simulink model "EZQStEnCtrl"  (R2018b)
settings: Solver=FixedStepDiscrete  StartTime=0.0  StopTime=10.0  FixedStep=0.01  RelTol=1e-3
undefined symbols (not defined in the file or in its folder): data, DrvStFtEn_Clear, DrvStFtEn_Set, PassStFtEn_Clear, PassStFtEn_Set, SecRwLtStArmScrnEn_Clear, SecRwLtStArmScrnEn_Set, SecRwLtStBkReclnEn_Clear, SecRwLtStBkReclnEn_Set, SecRwLtStFwdBkwdEn_Clear, SecRwLtStFwdBkwdEn_Set, SecRwLtStLgrstUpwdDnwdEn_Clear, SecRwLtStLgrstUpwdDnwdEn_Set, SecRwLtStLtwdRtwdEn_Clear, SecRwLtStLtwdRtwdEn_Set, SecRwRtStArmScrnEn_Clear, SecRwRtStArmScrnEn_Set, SecRwRtStBkReclnEn_Clear, SecRwRtStBkReclnEn_Set, SecRwRtStFwdBkwdEn_Clear, SecRwRtStFwdBkwdEn_Set, SecRwRtStLgrstUpwdDnwdEn_Clear, SecRwRtStLgrstUpwdDnwdEn_Set, SecRwRtStLtwdRtwdEn_Clear, SecRwRtStLtwdRtwdEn_Set
libraries: simulink x1
settings Model: Creator=sn2xws  LastModifiedBy=sn2xws
settings DataIOCC: SaveFormat=StructureWithTime
settings OptimizationCC: DefaultParameterBehavior=Inlined  EnhancedBackFolding=on  PassReuseOutputArgsAs=Individual arguments  ZeroExternalMemoryAtStartup=off  ZeroInternalMemoryAtStartup=off  OptimizeBlockOrder=speed  DifferentSizesBufferReuse=on  OptimizationCustomize=off
settings DebuggingCC: ParameterTunabilityLossMsg=error
settings ModelReferenceCC: ModelReferenceNumInstancesAllowed=Single
settings SFSimCC: MATLABDynamicMemAlloc=off
settings RTWCC: SystemTargetFile=autosar.tlc  GenCodeOnly=on  TemplateMakefile=ert_default_tmf  Description=AUTOSAR  GenerateReport=on  IncludeHyperlinkInReport=on  LaunchReport=on  GenerateTraceInfo=on  GenerateTraceReport=on  GenerateTraceReportSl=on  GenerateTraceReportSf=on  GenerateTraceReportEml=on  GenerateCodeMetricsReport=on
settings CodeAppCC: ForceParamTrailComments=on  IgnoreCustomStorageClasses=off  OperatorAnnotations=on  SimulinkDataObjDesc=on  SFDataObjDesc=on  InsertBlockDesc=on
settings STFCustomTargetCC: TargetLangStandard=C99 (ISO)  MultiwordLength=256  ParMdlRefBuildCompliant=on  CompOptLevelCompliant=on  IncludeMdlTerminateFcn=off  CombineOutputUpdateFcns=on  SuppressErrorStatus=on  ERTCustomFileBanners=on  SupportNonFinite=off  SupportComplex=off  SupportContinuousTime=off  SupportNonInlinedSFcns=off  RemoveResetFunc=on  MATLABClassNameForMDSCustomization=Simulink.SoftwareTarget.ERTCustomization  AutosarCompliant=on  UseToolchainInfoCompliant=on  LookupTableObjectStructAxisOrder=2,1,3,4,...  LUTObjectStructOrderEvenSpacing=Size,Table,Breakpoints  SystemTargetFile=autosar.tlc
settings ERTTargetCC: TargetLangStandard=C99 (ISO)  ConcurrentExecutionCompliant=off  IncludeMdlTerminateFcn=off  SuppressErrorStatus=on  SupportNonFinite=off  SupportComplex=off  ModelStepFunctionPrototypeControlCompliant=off  CPPClassGenCompliant=off  AutosarCompliant=on  LookupTableObjectStructAxisOrder=2,1,3,4,...  LUTObjectStructOrderEvenSpacing=Size,Table,Breakpoints  InlinedParameterPlacement=NonHierarchical  ERTCustomFileTemplate=example_file_process.tlc  ERTFilePackagingFormat=Compact

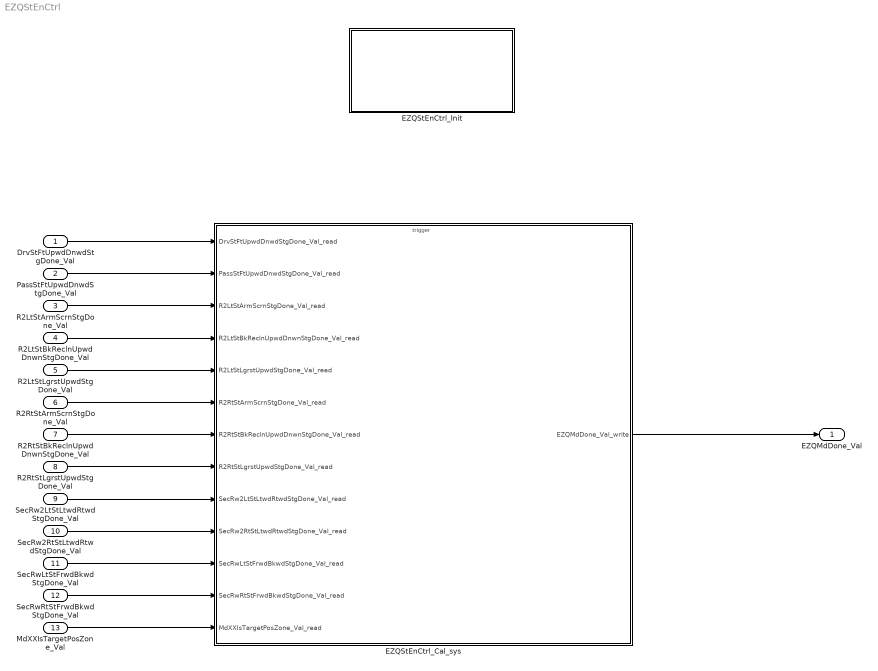
== system EZQStEnCtrl ==
  DrvStFtUpwdDnwdStgDone_Val : Inport  OutDataTypeStr=boolean  PortDimensions=1
  PassStFtUpwdDnwdStgDone_Val : Inport  Port=2  OutDataTypeStr=boolean  PortDimensions=1
  R2LtStArmScrnStgDone_Val : Inport  Port=3  OutDataTypeStr=boolean  PortDimensions=1
  R2LtStBkReclnUpwdDnwnStgDone_Val : Inport  Port=4  OutDataTypeStr=boolean  PortDimensions=1
  R2LtStLgrstUpwdStgDone_Val : Inport  Port=5  OutDataTypeStr=boolean  PortDimensions=1
  R2RtStArmScrnStgDone_Val : Inport  Port=6  OutDataTypeStr=boolean  PortDimensions=1
  R2RtStBkReclnUpwdDnwnStgDone_Val : Inport  Port=7  OutDataTypeStr=boolean  PortDimensions=1
  R2RtStLgrstUpwdStgDone_Val : Inport  Port=8  OutDataTypeStr=boolean  PortDimensions=1
  SecRw2LtStLtwdRtwdStgDone_Val : Inport  Port=9  OutDataTypeStr=boolean  PortDimensions=1
  SecRw2RtStLtwdRtwdStgDone_Val : Inport  Port=10  OutDataTypeStr=boolean  PortDimensions=1
  SecRwLtStFrwdBkwdStgDone_Val : Inport  Port=11  OutDataTypeStr=boolean  PortDimensions=1
  SecRwRtStFrwdBkwdStgDone_Val : Inport  Port=12  OutDataTypeStr=boolean  PortDimensions=1
  MdXXIsTargetPosZone_Val : Inport  Port=13  OutDataTypeStr=uint32  PortDimensions=1
  EZQStEnCtrl_Cal_sys : Subsystem
  EZQStEnCtrl_Init : Subsystem
  EZQMdDone_Val : Outport  OutDataTypeStr=uint8  PortDimensions=1
  wires:
  DrvStFtUpwdDnwdStgDone_Val/1 -> EZQStEnCtrl_Cal_sys/1(DrvStFtUpwdDnwdStgDone_Val_read)
  PassStFtUpwdDnwdStgDone_Val/1 -> EZQStEnCtrl_Cal_sys/2(PassStFtUpwdDnwdStgDone_Val_read)
  R2LtStArmScrnStgDone_Val/1 -> EZQStEnCtrl_Cal_sys/3(R2LtStArmScrnStgDone_Val_read)
  R2LtStBkReclnUpwdDnwnStgDone_Val/1 -> EZQStEnCtrl_Cal_sys/4(R2LtStBkReclnUpwdDnwnStgDone_Val_read)
  R2LtStLgrstUpwdStgDone_Val/1 -> EZQStEnCtrl_Cal_sys/5(R2LtStLgrstUpwdStgDone_Val_read)
  R2RtStArmScrnStgDone_Val/1 -> EZQStEnCtrl_Cal_sys/6(R2RtStArmScrnStgDone_Val_read)
  R2RtStBkReclnUpwdDnwnStgDone_Val/1 -> EZQStEnCtrl_Cal_sys/7(R2RtStBkReclnUpwdDnwnStgDone_Val_read)
  R2RtStLgrstUpwdStgDone_Val/1 -> EZQStEnCtrl_Cal_sys/8(R2RtStLgrstUpwdStgDone_Val_read)
  SecRw2LtStLtwdRtwdStgDone_Val/1 -> EZQStEnCtrl_Cal_sys/9(SecRw2LtStLtwdRtwdStgDone_Val_read)
  SecRw2RtStLtwdRtwdStgDone_Val/1 -> EZQStEnCtrl_Cal_sys/10(SecRw2RtStLtwdRtwdStgDone_Val_read)
  SecRwLtStFrwdBkwdStgDone_Val/1 -> EZQStEnCtrl_Cal_sys/11(SecRwLtStFrwdBkwdStgDone_Val_read)
  SecRwRtStFrwdBkwdStgDone_Val/1 -> EZQStEnCtrl_Cal_sys/12(SecRwRtStFrwdBkwdStgDone_Val_read)
  MdXXIsTargetPosZone_Val/1 -> EZQStEnCtrl_Cal_sys/13(MdXXIsTargetPosZone_Val_read)
  EZQStEnCtrl_Cal_sys/1(EZQMdDone_Val_write) -> EZQMdDone_Val/1

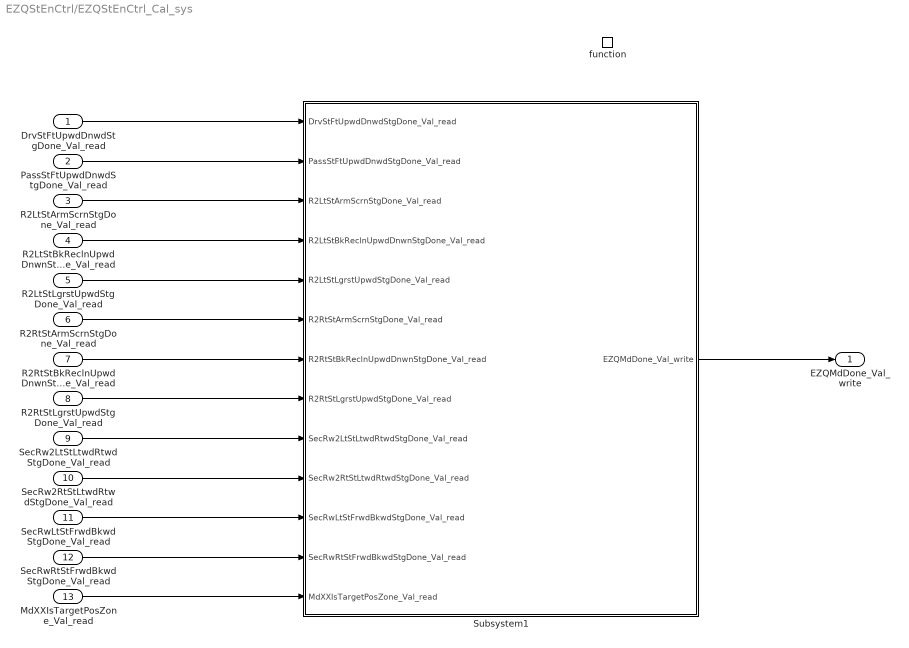
== system EZQStEnCtrl/EZQStEnCtrl_Cal_sys ==
  DrvStFtUpwdDnwdStgDone_Val_read : Inport
  PassStFtUpwdDnwdStgDone_Val_read : Inport  Port=2
  R2LtStArmScrnStgDone_Val_read : Inport  Port=3
  R2LtStBkReclnUpwdDnwnStgDone_Val_read : Inport  Port=4
  R2LtStLgrstUpwdStgDone_Val_read : Inport  Port=5
  R2RtStArmScrnStgDone_Val_read : Inport  Port=6
  R2RtStBkReclnUpwdDnwnStgDone_Val_read : Inport  Port=7
  R2RtStLgrstUpwdStgDone_Val_read : Inport  Port=8
  SecRw2LtStLtwdRtwdStgDone_Val_read : Inport  Port=9
  SecRw2RtStLtwdRtwdStgDone_Val_read : Inport  Port=10
  SecRwLtStFrwdBkwdStgDone_Val_read : Inport  Port=11
  SecRwRtStFrwdBkwdStgDone_Val_read : Inport  Port=12
  MdXXIsTargetPosZone_Val_read : Inport  Port=13
  function : TriggerPort  TriggerType=function-call  IsSimulinkFunction=on  FunctionName=EZQStEnCtrl_Cal  VariantControl=(inherit)
  Subsystem1 : Subsystem
  EZQMdDone_Val_write : Outport
      settings: EnsureOutportIsVirtual=on
  wires:
  Subsystem1/1(EZQMdDone_Val_write) -> EZQMdDone_Val_write/1
  DrvStFtUpwdDnwdStgDone_Val_read/1 -> Subsystem1/1(DrvStFtUpwdDnwdStgDone_Val_read)
  PassStFtUpwdDnwdStgDone_Val_read/1 -> Subsystem1/2(PassStFtUpwdDnwdStgDone_Val_read)
  R2LtStArmScrnStgDone_Val_read/1 -> Subsystem1/3(R2LtStArmScrnStgDone_Val_read)
  R2LtStBkReclnUpwdDnwnStgDone_Val_read/1 -> Subsystem1/4(R2LtStBkReclnUpwdDnwnStgDone_Val_read)
  R2LtStLgrstUpwdStgDone_Val_read/1 -> Subsystem1/5(R2LtStLgrstUpwdStgDone_Val_read)
  R2RtStArmScrnStgDone_Val_read/1 -> Subsystem1/6(R2RtStArmScrnStgDone_Val_read)
  R2RtStBkReclnUpwdDnwnStgDone_Val_read/1 -> Subsystem1/7(R2RtStBkReclnUpwdDnwnStgDone_Val_read)
  R2RtStLgrstUpwdStgDone_Val_read/1 -> Subsystem1/8(R2RtStLgrstUpwdStgDone_Val_read)
  SecRw2LtStLtwdRtwdStgDone_Val_read/1 -> Subsystem1/9(SecRw2LtStLtwdRtwdStgDone_Val_read)
  SecRw2RtStLtwdRtwdStgDone_Val_read/1 -> Subsystem1/10(SecRw2RtStLtwdRtwdStgDone_Val_read)
  SecRwLtStFrwdBkwdStgDone_Val_read/1 -> Subsystem1/11(SecRwLtStFrwdBkwdStgDone_Val_read)
  SecRwRtStFrwdBkwdStgDone_Val_read/1 -> Subsystem1/12(SecRwRtStFrwdBkwdStgDone_Val_read)
  MdXXIsTargetPosZone_Val_read/1 -> Subsystem1/13(MdXXIsTargetPosZone_Val_read)

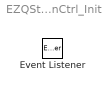
== system EZQStEnCtrl/EZQStEnCtrl_Init ==
  Event Listener : EventListener  EventName=reset

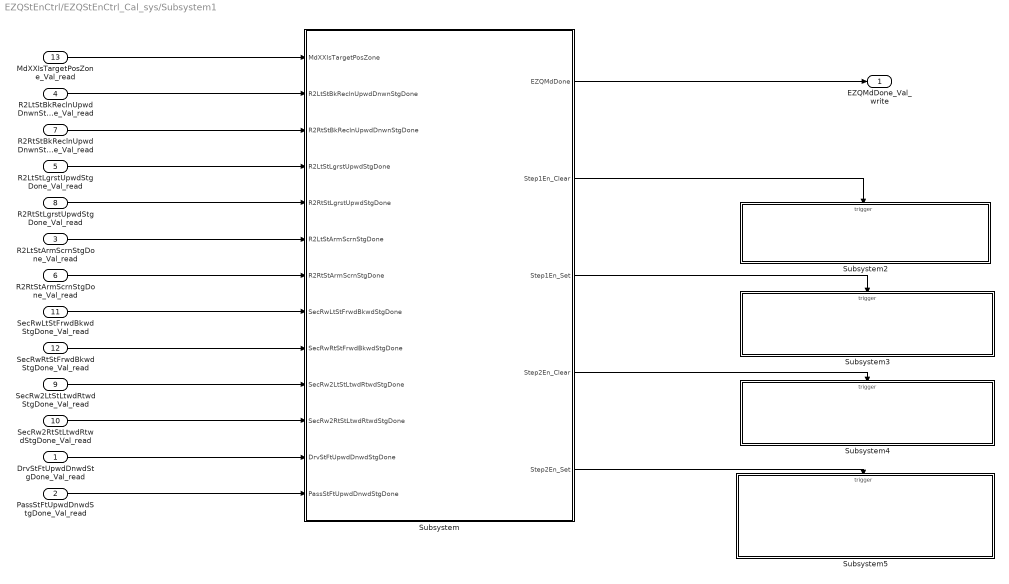
== system EZQStEnCtrl/EZQStEnCtrl_Cal_sys/Subsystem1 ==
  DrvStFtUpwdDnwdStgDone_Val_read : Inport
  PassStFtUpwdDnwdStgDone_Val_read : Inport  Port=2
  R2LtStArmScrnStgDone_Val_read : Inport  Port=3
  R2LtStBkReclnUpwdDnwnStgDone_Val_read : Inport  Port=4
  R2LtStLgrstUpwdStgDone_Val_read : Inport  Port=5
  R2RtStArmScrnStgDone_Val_read : Inport  Port=6
  R2RtStBkReclnUpwdDnwnStgDone_Val_read : Inport  Port=7
  R2RtStLgrstUpwdStgDone_Val_read : Inport  Port=8
  SecRw2LtStLtwdRtwdStgDone_Val_read : Inport  Port=9
  SecRw2RtStLtwdRtwdStgDone_Val_read : Inport  Port=10
  SecRwLtStFrwdBkwdStgDone_Val_read : Inport  Port=11
  SecRwRtStFrwdBkwdStgDone_Val_read : Inport  Port=12
  MdXXIsTargetPosZone_Val_read : Inport  Port=13
  Subsystem : Subsystem
  Subsystem2 : Subsystem
  Subsystem3 : Subsystem
  Subsystem4 : Subsystem
  Subsystem5 : Subsystem
  EZQMdDone_Val_write : Outport
      settings: EnsureOutportIsVirtual=on
  wires:
  PassStFtUpwdDnwdStgDone_Val_read/1 -> Subsystem/13(PassStFtUpwdDnwdStgDone)
  R2LtStLgrstUpwdStgDone_Val_read/1 -> Subsystem/4(R2LtStLgrstUpwdStgDone)
  Subsystem/1(EZQMdDone) -> EZQMdDone_Val_write/1
  DrvStFtUpwdDnwdStgDone_Val_read/1 -> Subsystem/12(DrvStFtUpwdDnwdStgDone)
  Subsystem/3(Step1En_Set) -> Subsystem3/Trigger
  SecRw2RtStLtwdRtwdStgDone_Val_read/1 -> Subsystem/11(SecRw2RtStLtwdRtwdStgDone)
  R2RtStBkReclnUpwdDnwnStgDone_Val_read/1 -> Subsystem/3(R2RtStBkReclnUpwdDnwnStgDone)
  R2LtStBkReclnUpwdDnwnStgDone_Val_read/1 -> Subsystem/2(R2LtStBkReclnUpwdDnwnStgDone)
  MdXXIsTargetPosZone_Val_read/1 -> Subsystem/1(MdXXIsTargetPosZone)
  R2RtStArmScrnStgDone_Val_read/1 -> Subsystem/7(R2RtStArmScrnStgDone)
  Subsystem/4(Step2En_Clear) -> Subsystem4/Trigger
  R2RtStLgrstUpwdStgDone_Val_read/1 -> Subsystem/5(R2RtStLgrstUpwdStgDone)
  SecRwLtStFrwdBkwdStgDone_Val_read/1 -> Subsystem/8(SecRwLtStFrwdBkwdStgDone)
  R2LtStArmScrnStgDone_Val_read/1 -> Subsystem/6(R2LtStArmScrnStgDone)
  Subsystem/2(Step1En_Clear) -> Subsystem2/Trigger
  SecRwRtStFrwdBkwdStgDone_Val_read/1 -> Subsystem/9(SecRwRtStFrwdBkwdStgDone)
  SecRw2LtStLtwdRtwdStgDone_Val_read/1 -> Subsystem/10(SecRw2LtStLtwdRtwdStgDone)
  Subsystem/5(Step2En_Set) -> Subsystem5/Trigger

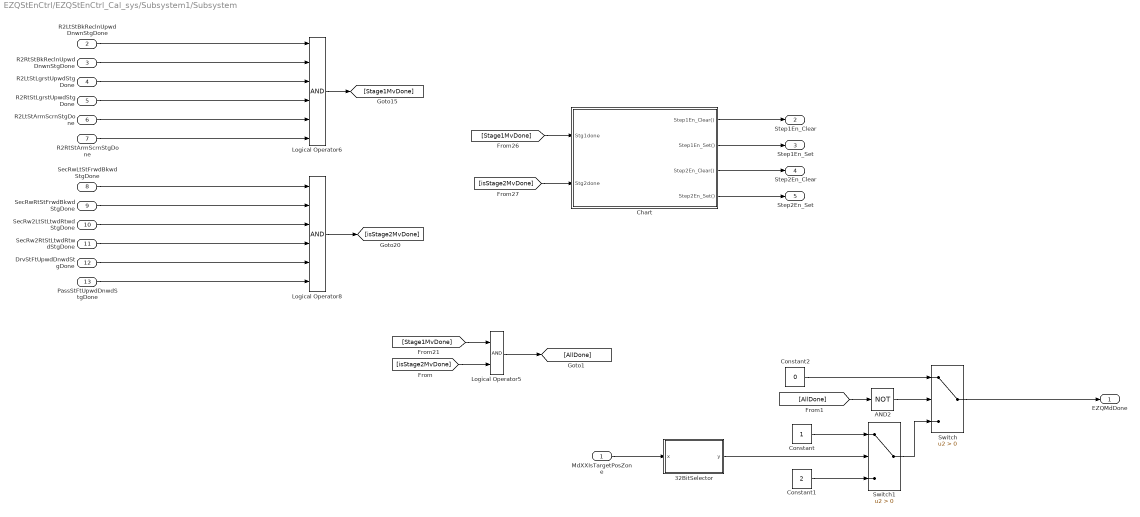
== system EZQStEnCtrl/EZQStEnCtrl_Cal_sys/Subsystem1/Subsystem ==
  MdXXIsTargetPosZone : Inport
  R2LtStBkReclnUpwdDnwnStgDone : Inport  Port=2
  R2RtStBkReclnUpwdDnwnStgDone : Inport  Port=3
  R2LtStLgrstUpwdStgDone : Inport  Port=4
  R2RtStLgrstUpwdStgDone : Inport  Port=5
  R2LtStArmScrnStgDone : Inport  Port=6
  R2RtStArmScrnStgDone : Inport  Port=7
  SecRwLtStFrwdBkwdStgDone : Inport  Port=8
  SecRwRtStFrwdBkwdStgDone : Inport  Port=9
  SecRw2LtStLtwdRtwdStgDone : Inport  Port=10
  SecRw2RtStLtwdRtwdStgDone : Inport  Port=11
  DrvStFtUpwdDnwdStgDone : Inport  Port=12
  PassStFtUpwdDnwdStgDone : Inport  Port=13
  32BitSelector : Subsystem  mask(32 Bit Selector){BitNum=3}
      mask prompts: BitNum "Select Bit Number"
      mask help: Allows selection of a particular bit (0-31) out of a packed word up to 32 bits long. Output will be true if the bit number selected via the mask parameter is equal to one.
      mask TypeOptions BitNum: 0 | 1 | 2 | 3 | 4 | 5 | 6 | 7 | 8 | 9 | 10 | 11 | 12 | 13 | 14 | 15 | 16 | 17 | 18 | 19 | 20 | 21 | 22 | 23 | 24 | 25 | 26 | 27 | 28 | 29 | 30 | 31
      mask Display:
      | text(0.5, 0.8,'BIT','horizontalAlignment','center')
      | text(0.5, 0.5,'SELECTOR','horizontalAlignment','center')
      | text(0.5, 0.2,['-- Bit ',char(get_param(gcb,'BitNum')),' --'],'horizontalAlignment','center')
  AND2 : Logic  Operator=NOT  AllPortsSameDT=off  OutDataTypeStr=boolean
  Chart : Stateflow chart  TreatAsAtomicUnit=on
  Constant : Constant  OutDataTypeStr=uint8
  Constant1 : Constant  Value=2  OutDataTypeStr=uint8
  Constant2 : Constant  Value=0  OutDataTypeStr=uint8
  Logical Operator5 : Logic  AllPortsSameDT=off  OutDataTypeStr=boolean
  Logical Operator6 : Logic  Inputs=6  AllPortsSameDT=off  OutDataTypeStr=boolean
  Logical Operator8 : Logic  Inputs=6  AllPortsSameDT=off  OutDataTypeStr=boolean
  Switch : Switch  Criteria=u2 > Threshold
  Switch1 : Switch  Criteria=u2 > Threshold
  EZQMdDone : Outport
  Step1En_Clear : Outport  Port=2
  Step1En_Set : Outport  Port=3
  Step2En_Clear : Outport  Port=4
  Step2En_Set : Outport  Port=5
  wires:
  [isStage2MvDone] -> Logical Operator5/2
  SecRwRtStFrwdBkwdStgDone/1 -> Logical Operator8/2
  R2LtStBkReclnUpwdDnwnStgDone/1 -> Logical Operator6/1
  R2RtStBkReclnUpwdDnwnStgDone/1 -> Logical Operator6/2
  [isStage2MvDone] -> Chart/2(Stg2done)
  Logical Operator6/1 -> [Stage1MvDone]
  [AllDone] -> AND2/1
  MdXXIsTargetPosZone/1 -> 32BitSelector/1(x)
  R2LtStArmScrnStgDone/1 -> Logical Operator6/5
  [Stage1MvDone] -> Logical Operator5/1
  [Stage1MvDone] -> Chart/1(Stg1done)
  R2RtStLgrstUpwdStgDone/1 -> Logical Operator6/4
  Logical Operator5/1 -> [AllDone]
  SecRw2LtStLtwdRtwdStgDone/1 -> Logical Operator8/3
  R2LtStLgrstUpwdStgDone/1 -> Logical Operator6/3
  Logical Operator8/1 -> [isStage2MvDone]
  SecRwLtStFrwdBkwdStgDone/1 -> Logical Operator8/1
  R2RtStArmScrnStgDone/1 -> Logical Operator6/6
  SecRw2RtStLtwdRtwdStgDone/1 -> Logical Operator8/4
  PassStFtUpwdDnwdStgDone/1 -> Logical Operator8/6
  DrvStFtUpwdDnwdStgDone/1 -> Logical Operator8/5
  Switch1/1 -> Switch/3
  Switch/1 -> EZQMdDone/1
  Chart/1(Step1En_Clear()) -> Step1En_Clear/1
  Chart/2(Step1En_Set()) -> Step1En_Set/1
  Chart/3(Step2En_Clear()) -> Step2En_Clear/1
  Chart/4(Step2En_Set()) -> Step2En_Set/1
  Constant/1 -> Switch1/1
  Constant1/1 -> Switch1/3
  Constant2/1 -> Switch/1
  AND2/1 -> Switch/2
  32BitSelector/1(y) -> Switch1/2

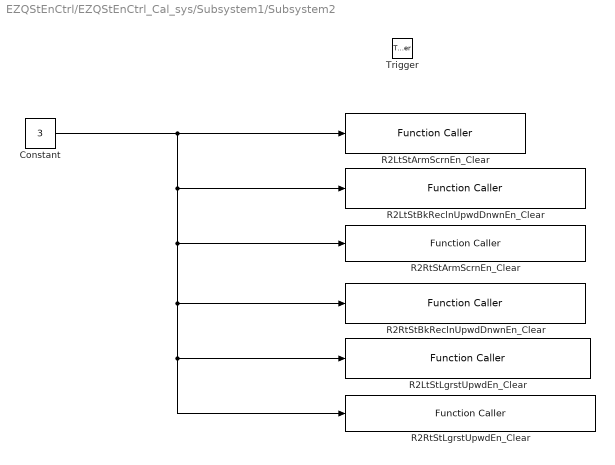
== system EZQStEnCtrl/EZQStEnCtrl_Cal_sys/Subsystem1/Subsystem2 ==
  Trigger : TriggerPort  TriggerType=function-call  VariantControl=Variant  PortDimensions=1
  Constant : Constant  Value=3  OutDataTypeStr=uint8
  R2LtStArmScrnEn_Clear : FunctionCaller  FunctionPrototype=SecRwLtStArmScrnEn_Clear(data)  InputArgumentSpecifications=uint8(1)
  R2LtStBkReclnUpwdDnwnEn_Clear : FunctionCaller  FunctionPrototype=SecRwLtStBkReclnEn_Clear(data)  InputArgumentSpecifications=uint8(1)
  R2LtStLgrstUpwdEn_Clear : FunctionCaller  FunctionPrototype=SecRwLtStLgrstUpwdDnwdEn_Clear(data)  InputArgumentSpecifications=uint8(1)
  R2RtStArmScrnEn_Clear : FunctionCaller  FunctionPrototype=SecRwRtStArmScrnEn_Clear(data)  InputArgumentSpecifications=uint8(1)
  R2RtStBkReclnUpwdDnwnEn_Clear : FunctionCaller  FunctionPrototype=SecRwRtStBkReclnEn_Clear(data)  InputArgumentSpecifications=uint8(1)
  R2RtStLgrstUpwdEn_Clear : FunctionCaller  FunctionPrototype=SecRwRtStLgrstUpwdDnwdEn_Clear(data)  InputArgumentSpecifications=uint8(1)
  wires:
  Constant/1 -> R2RtStArmScrnEn_Clear/1, R2RtStBkReclnUpwdDnwnEn_Clear/1, R2RtStLgrstUpwdEn_Clear/1, R2LtStLgrstUpwdEn_Clear/1, R2LtStBkReclnUpwdDnwnEn_Clear/1, R2LtStArmScrnEn_Clear/1

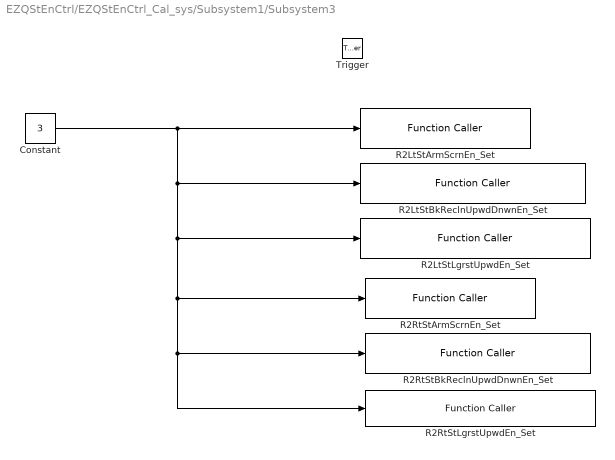
== system EZQStEnCtrl/EZQStEnCtrl_Cal_sys/Subsystem1/Subsystem3 ==
  Trigger : TriggerPort  TriggerType=function-call  VariantControl=Variant  PortDimensions=1
  Constant : Constant  Value=3  OutDataTypeStr=uint8
  R2LtStArmScrnEn_Set : FunctionCaller  FunctionPrototype=SecRwLtStArmScrnEn_Set(data)  InputArgumentSpecifications=uint8(1)
  R2LtStBkReclnUpwdDnwnEn_Set : FunctionCaller  FunctionPrototype=SecRwLtStBkReclnEn_Set(data)  InputArgumentSpecifications=uint8(1)
  R2LtStLgrstUpwdEn_Set : FunctionCaller  FunctionPrototype=SecRwLtStLgrstUpwdDnwdEn_Set(data)  InputArgumentSpecifications=uint8(1)
  R2RtStArmScrnEn_Set : FunctionCaller  FunctionPrototype=SecRwRtStArmScrnEn_Set(data)  InputArgumentSpecifications=uint8(1)
  R2RtStBkReclnUpwdDnwnEn_Set : FunctionCaller  FunctionPrototype=SecRwRtStBkReclnEn_Set(data)  InputArgumentSpecifications=uint8(1)
  R2RtStLgrstUpwdEn_Set : FunctionCaller  FunctionPrototype=SecRwRtStLgrstUpwdDnwdEn_Set(data)  InputArgumentSpecifications=uint8(1)
  wires:
  Constant/1 -> R2LtStArmScrnEn_Set/1, R2LtStBkReclnUpwdDnwnEn_Set/1, R2LtStLgrstUpwdEn_Set/1, R2RtStArmScrnEn_Set/1, R2RtStBkReclnUpwdDnwnEn_Set/1, R2RtStLgrstUpwdEn_Set/1

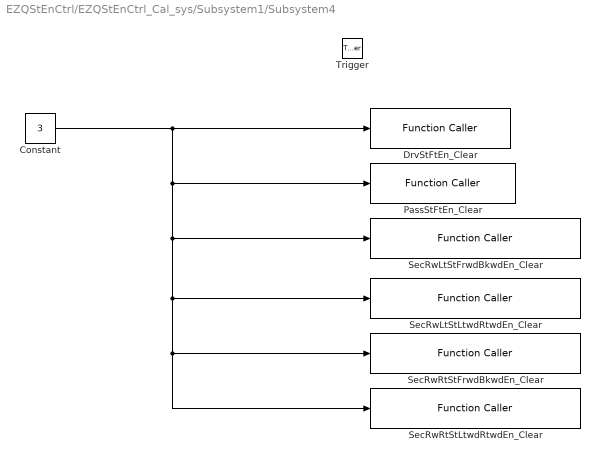
== system EZQStEnCtrl/EZQStEnCtrl_Cal_sys/Subsystem1/Subsystem4 ==
  Trigger : TriggerPort  TriggerType=function-call  VariantControl=Variant  PortDimensions=1
  Constant : Constant  Value=3  OutDataTypeStr=uint8
  DrvStFtEn_Clear : FunctionCaller  FunctionPrototype=DrvStFtEn_Clear(data)  InputArgumentSpecifications=uint8(1)
  PassStFtEn_Clear : FunctionCaller  FunctionPrototype=PassStFtEn_Clear(data)  InputArgumentSpecifications=uint8(1)
  SecRwLtStFrwdBkwdEn_Clear : FunctionCaller  FunctionPrototype=SecRwLtStFwdBkwdEn_Clear(data)  InputArgumentSpecifications=uint8(1)
  SecRwLtStLtwdRtwdEn_Clear : FunctionCaller  FunctionPrototype=SecRwLtStLtwdRtwdEn_Clear(data)  InputArgumentSpecifications=uint8(1)
  SecRwRtStFrwdBkwdEn_Clear : FunctionCaller  FunctionPrototype=SecRwRtStFwdBkwdEn_Clear(data)  InputArgumentSpecifications=uint8(1)
  SecRwRtStLtwdRtwdEn_Clear : FunctionCaller  FunctionPrototype=SecRwRtStLtwdRtwdEn_Clear(data)  InputArgumentSpecifications=uint8(1)
  wires:
  Constant/1 -> DrvStFtEn_Clear/1, PassStFtEn_Clear/1, SecRwLtStFrwdBkwdEn_Clear/1, SecRwLtStLtwdRtwdEn_Clear/1, SecRwRtStLtwdRtwdEn_Clear/1, SecRwRtStFrwdBkwdEn_Clear/1

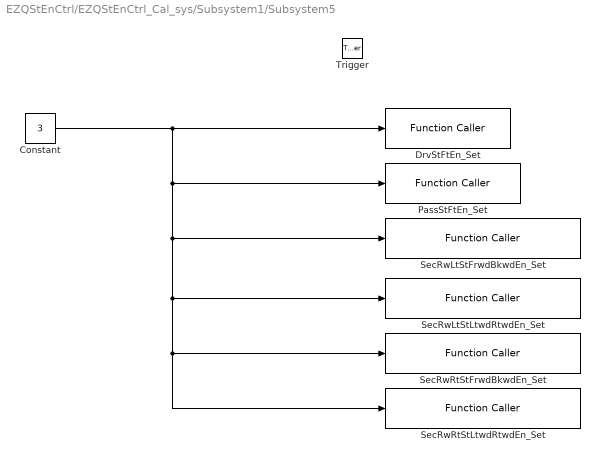
== system EZQStEnCtrl/EZQStEnCtrl_Cal_sys/Subsystem1/Subsystem5 ==
  Trigger : TriggerPort  TriggerType=function-call  VariantControl=Variant  PortDimensions=1
  Constant : Constant  Value=3  OutDataTypeStr=uint8
  DrvStFtEn_Set : FunctionCaller  FunctionPrototype=DrvStFtEn_Set(data)  InputArgumentSpecifications=uint8(1)
  PassStFtEn_Set : FunctionCaller  FunctionPrototype=PassStFtEn_Set(data)  InputArgumentSpecifications=uint8(1)
  SecRwLtStFrwdBkwdEn_Set : FunctionCaller  FunctionPrototype=SecRwLtStFwdBkwdEn_Set(data)  InputArgumentSpecifications=uint8(1)
  SecRwLtStLtwdRtwdEn_Set : FunctionCaller  FunctionPrototype=SecRwLtStLtwdRtwdEn_Set(data)  InputArgumentSpecifications=uint8(1)
  SecRwRtStFrwdBkwdEn_Set : FunctionCaller  FunctionPrototype=SecRwRtStFwdBkwdEn_Set(data)  InputArgumentSpecifications=uint8(1)
  SecRwRtStLtwdRtwdEn_Set : FunctionCaller  FunctionPrototype=SecRwRtStLtwdRtwdEn_Set(data)  InputArgumentSpecifications=uint8(1)
  wires:
  Constant/1 -> DrvStFtEn_Set/1, PassStFtEn_Set/1, SecRwLtStFrwdBkwdEn_Set/1, SecRwLtStLtwdRtwdEn_Set/1, SecRwRtStLtwdRtwdEn_Set/1, SecRwRtStFrwdBkwdEn_Set/1

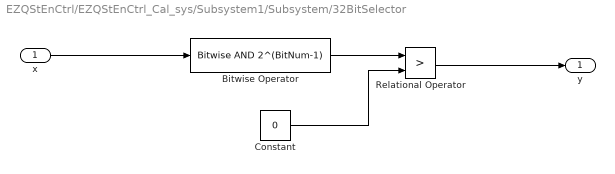
== system EZQStEnCtrl/EZQStEnCtrl_Cal_sys/Subsystem1/Subsystem/32BitSelector ==
  x : Inport
  Bitwise Operator : simulink/Logic and Bit Operations/Bitwise Operator  logicop=AND  UseBitMask=on  BitMask=2^(BitNum-1)  BitMaskRealWorld=Stored Integer
  Constant : Constant  Value=0  OutDataTypeStr=uint32
  Relational Operator : RelationalOperator  Operator=>  OutDataTypeStr=boolean  RndMeth=Simplest
  y : Outport
  wires:
  Relational Operator/1 -> y/1
  Constant/1 -> Relational Operator/2
  x/1 -> Bitwise Operator/1
  Bitwise Operator/1 -> Relational Operator/1

== stateflow chart EZQStEnCtrl/EZQStEnCtrl_Cal_sys/Subsystem1/Subsystem/Chart ==
  (default) -> (junction 31)
  (junction 31) -> (junction 34) [order 1] : [!Stg1done]
  (junction 31) -> (junction 38) [order 2]
  (junction 34) -> (junction 47) : {
      | Step1En_Set;
      | Step2En_Clear;
      | }
  (junction 38) -> (junction 24) [order 1] : [!Stg2done]
  (junction 38) -> (junction 71) [order 2] : {
      | Step1En_Clear;
      | Step2En_Clear;
      | }
  (junction 24) -> (junction 72) : {
      | Step1En_Clear;
      | Step2En_Set;
      | }
  (junction 72) -> (junction 71)
  (junction 47) -> (junction 72)
  (junction 71) -> (junction 48)
  data: Stg1done input boolean; Stg2done input boolean
  events: Step1En_Clear output FUNCTION_CALL_EVENT; Step1En_Set output FUNCTION_CALL_EVENT; Step2En_Clear output FUNCTION_CALL_EVENT; Step2En_Set output FUNCTION_CALL_EVENT
